simulink model "lab52"  (R2018b)
settings: Solver=VariableStepAuto  StartTime=0.0  StopTime=0.8  MaxStep=1e-3  RelTol=1e-3
settings Model: Creator=wangh  LastModifiedBy=wangh

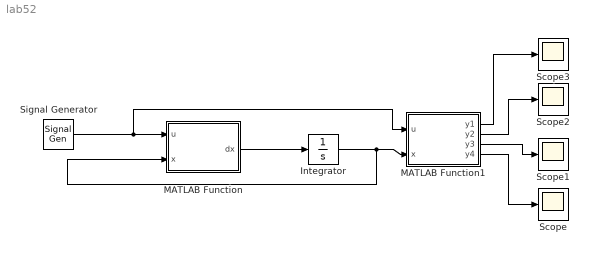
== system lab52 ==
  Integrator : Integrator
  MATLAB Function : MATLAB Function  TreatAsAtomicUnit=on
  MATLAB Function1 : MATLAB Function  TreatAsAtomicUnit=on
  Scope{,1..3} (4 alike) : Scope
  Signal Generator : SignalGenerator  Amplitude=120  Frequency=2*pi*60  Units=rad/sec
  wires:
  Signal Generator/1 -> MATLAB Function1/1(u), MATLAB Function/1(u)
  MATLAB Function/1(dx) -> Integrator/1
  Integrator/1 -> MATLAB Function/2(x), MATLAB Function1/2(x)
  MATLAB Function1/4(y4) -> Scope/1
  MATLAB Function1/3(y3) -> Scope1/1
  MATLAB Function1/2(y2) -> Scope2/1
  MATLAB Function1/1(y1) -> Scope3/1

== matlab function lab52/MATLAB Function1 ==
  data: u input; y1 output; x input; y2 output; y3 output; y4 output
function [y1,y2,y3,y4] = fcn2(u,x)
[R,~,~,N]=def();
y1 = R*x(4);
y2 = x(1);
y3 = u/N-x(1);
y4 = diode(u/N-x(1));
end

== matlab function lab52/MATLAB Function ==
  data: u input; dx output; x input
function dx = fcn(u,x)
[R,C,L,N]=def();  
dx = zeros(4,1);
dx(1) = (diode(u/N-x(1))-x(3))/C;
dx(2) = (x(3)-x(4))/C;
dx(3) = (x(1)-x(2))/L;
dx(4) = (x(2)-x(4)*R)/L;

end
